simulink model "control_lvlh_sim"  (R2023b)
settings: Solver=ode5  StartTime=0.0  StopTime=10000  RelTol=1e-3
values from neighbouring files (symbols this model uses):
  a = 6.851221970532768e+03    (= 6851.22197053)    [complete_model.m]    (also in control_lvlh.m; lvlh_control.m; untitled.m)
  alpha1 = 0.4    [complete_model.m]    (also in control_lvlh.m; lvlh_control.m; untitled.m)
  alpha2 = 0.1    [complete_model.m]    (also in control_lvlh.m; lvlh_control.m; untitled.m)
  alpha3 = 0.5    [complete_model.m]    (also in control_lvlh.m; lvlh_control.m; untitled.m)
  D = zeros(3)    [complete_model.m]    (also in control_lvlh.m; lvlh_control.m = zeros(3,3); untitled.m = zeros(3,3))
  e = 0    [complete_model.m]    (also in control_lvlh.m; lvlh_control.m; untitled.m)
  FOV_earth = deg2rad(33)    [complete_model.m]    (also in control_lvlh.m; lvlh_control.m; untitled.m)
  FOV_sun = deg2rad(85)    [control_lvlh.m]    (also in lvlh_control.m; untitled.m)
  freq_earth = 30    [complete_model.m]    (also in control_lvlh.m = 5; lvlh_control.m = 5; untitled.m = 5)
  freq_mag = 30    [complete_model.m]    (also in control_lvlh.m = 5; lvlh_control.m = 5; untitled.m = 5)
  freq_sun = 30    [complete_model.m]    (also in control_lvlh.m = 5; lvlh_control.m = 5; untitled.m = 5)
  H0 = sqrt(g01^2+g11^2+h11^2)*1e-9    [complete_model.m]    (also in control_lvlh.m; lvlh_control.m; untitled.m)
  I = diag([I1 I2 I3])    [complete_model.m]    (also in control_lvlh.m; lvlh_control.m; untitled.m)
  Iinv = I\eye(3)    [complete_model.m]    (also in control_lvlh.m; lvlh_control.m; untitled.m)
  incl = deg2rad(11.5)    [complete_model.m]    (also in control_lvlh.m; lvlh_control.m; untitled.m)
  jb = [0.01; 0.05; 0.01]    [complete_model.m]    (also in control_lvlh.m; lvlh_control.m; untitled.m)
  K = place(A,B,p)    [complete_model.m]    (also in control_lvlh.m = [Kd Kp]; lvlh_control.m = 1/100*K)
  k_gain = (4*pi/T) * (1 + sin(chsi)) * I2    [complete_model.m]    (also in control_lvlh.m)
  max_dip = 15    [complete_model.m]    (also in control_lvlh.m = 150; lvlh_control.m = 150; untitled.m = 150)
  mu = astroConstants(13)    [complete_model.m]    (also in control_lvlh.m; lvlh_control.m; untitled.m)
  n = sqrt(mu/a^3)    [complete_model.m]    (also in control_lvlh.m; lvlh_control.m; untitled.m)
  omega0 = 0.06 * rand(3,1)    [complete_model.m]    (also in control_lvlh.m = [0; 0; n]; lvlh_control.m = [0; 0; n]; untitled.m = [0; 0; n])
  omegaE = deg2rad(15)/3600    [complete_model.m]    (also in control_lvlh.m; lvlh_control.m; untitled.m)
  rs = -rr    [complete_model.m]    (also in control_lvlh.m; lvlh_control.m; untitled.m)
  Rt = astroConstants(23)    [complete_model.m]    (also in control_lvlh.m; lvlh_control.m; untitled.m)
  s0 = 2*pi*rand(3,1)    [complete_model.m]    (also in control_lvlh.m = [2.099, -0.2003, -1.703]; lvlh_control.m = [2.099, -0.2003, -1.703]; untitled.m = [2.099, -0.2003, -1.703])
  tol = 0.2    [complete_model.m]    (also in control_lvlh.m; lvlh_control.m; untitled.m)
undefined symbols (not defined in the file or in its folder): magnitude
libraries: matrix_library x9, vrlib x9, simulink x8, sharedutil x2, cstblocks x2, dspmathops x2, dspfactors x1, aerolibutil x1
(part 2 of 2)

== system control_lvlh_sim/Kinematics/Kinematics 312/s_313 - A/R1 ==
  x : Inport
  Constant : Constant  Value=[1; 0; 0]
  Constant1 : Constant  Value=0
  Cos : Trigonometry  Operator=cos
  Gain : Gain  Gain=-1
  Matrix Concatenate : Concatenate  NumInputs=3  Mode=Multidimensional array  ConcatenateDimension=2
  Sin : Trigonometry
  Vector Concatenate : Concatenate  NumInputs=3
  Vector Concatenate1 : Concatenate  NumInputs=3
  R1 : Outport
  wires:
  Sin/1 -> Gain/1, Vector Concatenate/2
  Gain/1 -> Vector Concatenate1/3
  Cos/1 -> Vector Concatenate1/2, Vector Concatenate/3
  Constant1/1 -> Vector Concatenate1/1, Vector Concatenate/1
  Vector Concatenate/1 -> Matrix Concatenate/3
  Constant/1 -> Matrix Concatenate/1
  Vector Concatenate1/1 -> Matrix Concatenate/2
  x/1 -> Sin/1, Cos/1
  Matrix Concatenate/1 -> R1/1

== system control_lvlh_sim/Kinematics/Kinematics 312/s_313 - A/R3_1 ==
  x : Inport
  Constant : Constant  Value=[0; 0; 1]
  Constant1 : Constant  Value=0
  Cos : Trigonometry  Operator=cos
  Gain : Gain  Gain=-1
  Matrix Concatenate : Concatenate  NumInputs=3  Mode=Multidimensional array  ConcatenateDimension=2
  Sin : Trigonometry
  Vector Concatenate : Concatenate  NumInputs=3
  Vector Concatenate1 : Concatenate  NumInputs=3
  R3 : Outport
  wires:
  Matrix Concatenate/1 -> R3/1
  Constant1/1 -> Vector Concatenate1/3, Vector Concatenate/3
  x/1 -> Cos/1, Sin/1
  Vector Concatenate1/1 -> Matrix Concatenate/2
  Gain/1 -> Vector Concatenate/2
  Constant/1 -> Matrix Concatenate/3
  Cos/1 -> Vector Concatenate/1, Vector Concatenate1/2
  Sin/1 -> Gain/1, Vector Concatenate1/1
  Vector Concatenate/1 -> Matrix Concatenate/1

== system control_lvlh_sim/Kinematics/Kinematics 312/s_313 - A/R3_2 ==
  x : Inport
  Constant : Constant  Value=[0; 0; 1]
  Constant1 : Constant  Value=0
  Cos : Trigonometry  Operator=cos
  Gain : Gain  Gain=-1
  Matrix Concatenate : Concatenate  NumInputs=3  Mode=Multidimensional array  ConcatenateDimension=2
  Sin : Trigonometry
  Vector Concatenate : Concatenate  NumInputs=3
  Vector Concatenate1 : Concatenate  NumInputs=3
  R3 : Outport
  wires:
  Vector Concatenate/1 -> Matrix Concatenate/1
  Sin/1 -> Vector Concatenate1/1, Gain/1
  Cos/1 -> Vector Concatenate1/2, Vector Concatenate/1
  Constant/1 -> Matrix Concatenate/3
  Gain/1 -> Vector Concatenate/2
  Vector Concatenate1/1 -> Matrix Concatenate/2
  x/1 -> Sin/1, Cos/1
  Constant1/1 -> Vector Concatenate/3, Vector Concatenate1/3
  Matrix Concatenate/1 -> R3/1

== system control_lvlh_sim/Kinematics/Kinematics 313/Euler angles/Subsystem ==
  In1 : Inport
  In2 : Inport  Port=2
  In3 : Inport  Port=3
  Cos : Trigonometry  Operator=cos
  Product : Product
  Product1 : Product
  Sin : Trigonometry
  Sum : Sum
  Out1 : Outport
  wires:
  Sum/1 -> Out1/1
  Product1/1 -> Sum/2
  Product/1 -> Sum/1
  In2/1 -> Product1/2
  Sin/1 -> Product1/1
  Cos/1 -> Product/2
  In1/1 -> Product/1
  In3/1 -> Cos/1, Sin/1

== system control_lvlh_sim/Kinematics/Kinematics 313/Euler angles/Subsystem1 ==
  In1 : Inport
  In2 : Inport  Port=2
  In3 : Inport  Port=3
  Cos : Trigonometry  Operator=cos
  Product : Product
  Product1 : Product
  Sin : Trigonometry
  Sum : Sum
  Out1 : Outport
  wires:
  In3/1 -> Sin/1, Cos/1
  In1/1 -> Product/1
  Cos/1 -> Product/2
  Sin/1 -> Product1/1
  In2/1 -> Product1/2
  Product/1 -> Sum/1
  Product1/1 -> Sum/2
  Sum/1 -> Out1/1

== system control_lvlh_sim/Kinematics/Kinematics 313/Euler angles/Subsystem2 ==
  In1 : Inport
  In2 : Inport  Port=2
  In3 : Inport  Port=3
  Cos : Trigonometry  Operator=cos
  Product : Product
  Product1 : Product
  Sin : Trigonometry
  Sum : Sum
  Out1 : Outport
  wires:
  Sum/1 -> Out1/1
  Product1/1 -> Sum/2
  Product/1 -> Sum/1
  In2/1 -> Product1/2
  Sin/1 -> Product1/1
  Cos/1 -> Product/2
  In1/1 -> Product/1
  In3/1 -> Cos/1, Sin/1

== system control_lvlh_sim/Kinematics/Kinematics 313/s_312 - A/R1 ==
  x : Inport
  Constant : Constant  Value=[1; 0; 0]
  Constant1 : Constant  Value=0
  Cos : Trigonometry  Operator=cos
  Gain : Gain  Gain=-1
  Matrix Concatenate : Concatenate  NumInputs=3  Mode=Multidimensional array  ConcatenateDimension=2
  Sin : Trigonometry
  Vector Concatenate : Concatenate  NumInputs=3
  Vector Concatenate1 : Concatenate  NumInputs=3
  R1 : Outport
  wires:
  Matrix Concatenate/1 -> R1/1
  x/1 -> Cos/1, Sin/1
  Vector Concatenate1/1 -> Matrix Concatenate/2
  Constant/1 -> Matrix Concatenate/1
  Vector Concatenate/1 -> Matrix Concatenate/3
  Constant1/1 -> Vector Concatenate/1, Vector Concatenate1/1
  Cos/1 -> Vector Concatenate/3, Vector Concatenate1/2
  Gain/1 -> Vector Concatenate1/3
  Sin/1 -> Vector Concatenate/2, Gain/1

== system control_lvlh_sim/Kinematics/Kinematics 313/s_312 - A/R2 ==
  x : Inport
  Constant : Constant  Value=[0; 1; 0]
  Constant1 : Constant  Value=0
  Cos : Trigonometry  Operator=cos
  Gain : Gain  Gain=-1
  Matrix Concatenate : Concatenate  NumInputs=3  Mode=Multidimensional array  ConcatenateDimension=2
  Sin : Trigonometry
  Vector Concatenate : Concatenate  NumInputs=3
  Vector Concatenate1 : Concatenate  NumInputs=3
  R2 : Outport
  wires:
  Vector Concatenate/1 -> Matrix Concatenate/1
  x/1 -> Sin/1, Cos/1
  Matrix Concatenate/1 -> R2/1
  Constant/1 -> Matrix Concatenate/2
  Vector Concatenate1/1 -> Matrix Concatenate/3
  Constant1/1 -> Vector Concatenate/2, Vector Concatenate1/2
  Cos/1 -> Vector Concatenate1/3, Vector Concatenate/1
  Sin/1 -> Gain/1, Vector Concatenate/3
  Gain/1 -> Vector Concatenate1/1

== system control_lvlh_sim/Kinematics/Kinematics 313/s_312 - A/R3 ==
  x : Inport
  Constant : Constant  Value=[0; 0; 1]
  Constant1 : Constant  Value=0
  Cos : Trigonometry  Operator=cos
  Gain : Gain  Gain=-1
  Matrix Concatenate : Concatenate  NumInputs=3  Mode=Multidimensional array  ConcatenateDimension=2
  Sin : Trigonometry
  Vector Concatenate : Concatenate  NumInputs=3
  Vector Concatenate1 : Concatenate  NumInputs=3
  R3 : Outport
  wires:
  Vector Concatenate/1 -> Matrix Concatenate/1
  Sin/1 -> Vector Concatenate1/1, Gain/1
  Cos/1 -> Vector Concatenate1/2, Vector Concatenate/1
  Constant/1 -> Matrix Concatenate/3
  Gain/1 -> Vector Concatenate/2
  Vector Concatenate1/1 -> Matrix Concatenate/2
  x/1 -> Sin/1, Cos/1
  Constant1/1 -> Vector Concatenate/3, Vector Concatenate1/3
  Matrix Concatenate/1 -> R3/1

== system control_lvlh_sim/Kinematics/Kinematics 313/s_313 - A/R1 ==
  x : Inport
  Constant : Constant  Value=[1; 0; 0]
  Constant1 : Constant  Value=0
  Cos : Trigonometry  Operator=cos
  Gain : Gain  Gain=-1
  Matrix Concatenate : Concatenate  NumInputs=3  Mode=Multidimensional array  ConcatenateDimension=2
  Sin : Trigonometry
  Vector Concatenate : Concatenate  NumInputs=3
  Vector Concatenate1 : Concatenate  NumInputs=3
  R1 : Outport
  wires:
  Sin/1 -> Gain/1, Vector Concatenate/2
  Gain/1 -> Vector Concatenate1/3
  Cos/1 -> Vector Concatenate1/2, Vector Concatenate/3
  Constant1/1 -> Vector Concatenate1/1, Vector Concatenate/1
  Vector Concatenate/1 -> Matrix Concatenate/3
  Constant/1 -> Matrix Concatenate/1
  Vector Concatenate1/1 -> Matrix Concatenate/2
  x/1 -> Sin/1, Cos/1
  Matrix Concatenate/1 -> R1/1

== system control_lvlh_sim/Kinematics/Kinematics 313/s_313 - A/R3_1 ==
  x : Inport
  Constant : Constant  Value=[0; 0; 1]
  Constant1 : Constant  Value=0
  Cos : Trigonometry  Operator=cos
  Gain : Gain  Gain=-1
  Matrix Concatenate : Concatenate  NumInputs=3  Mode=Multidimensional array  ConcatenateDimension=2
  Sin : Trigonometry
  Vector Concatenate : Concatenate  NumInputs=3
  Vector Concatenate1 : Concatenate  NumInputs=3
  R3 : Outport
  wires:
  Matrix Concatenate/1 -> R3/1
  Constant1/1 -> Vector Concatenate1/3, Vector Concatenate/3
  x/1 -> Cos/1, Sin/1
  Vector Concatenate1/1 -> Matrix Concatenate/2
  Gain/1 -> Vector Concatenate/2
  Constant/1 -> Matrix Concatenate/3
  Cos/1 -> Vector Concatenate/1, Vector Concatenate1/2
  Sin/1 -> Gain/1, Vector Concatenate1/1
  Vector Concatenate/1 -> Matrix Concatenate/1

== system control_lvlh_sim/Kinematics/Kinematics 313/s_313 - A/R3_2 ==
  x : Inport
  Constant : Constant  Value=[0; 0; 1]
  Constant1 : Constant  Value=0
  Cos : Trigonometry  Operator=cos
  Gain : Gain  Gain=-1
  Matrix Concatenate : Concatenate  NumInputs=3  Mode=Multidimensional array  ConcatenateDimension=2
  Sin : Trigonometry
  Vector Concatenate : Concatenate  NumInputs=3
  Vector Concatenate1 : Concatenate  NumInputs=3
  R3 : Outport
  wires:
  Vector Concatenate/1 -> Matrix Concatenate/1
  Sin/1 -> Vector Concatenate1/1, Gain/1
  Cos/1 -> Vector Concatenate1/2, Vector Concatenate/1
  Constant/1 -> Matrix Concatenate/3
  Gain/1 -> Vector Concatenate/2
  Vector Concatenate1/1 -> Matrix Concatenate/2
  x/1 -> Sin/1, Cos/1
  Constant1/1 -> Vector Concatenate/3, Vector Concatenate1/3
  Matrix Concatenate/1 -> R3/1
